simulink model "L0401"  (Simulink 9.1)
settings: Solver=ode5  StartTime=0.0  StopTime=100  FixedStep=0.001  RelTol=1e-3
values from neighbouring files (symbols this model uses):
  c = input('Damping parameter c= ')    [vehicle.m]
  hole_depth = 0.15    [vehicle.m]
  k = input('Spring stiffness k= ')    [vehicle.m]
  m = 1000    [vehicle.m]
  t1 = hole_start/v    (= 22.5)    [vehicle.m]
  t2 = (hole_start + hole_width)/v    (= 22.55)    [vehicle.m]
settings Model: Creator=Asus  LastModifiedBy=Asus
settings DataIOCC: SaveFormat=Dataset
settings OptimizationCC: LifeSpan=auto
settings DebuggingCC: UnderspecifiedInitializationDetection=Simplified  MergeDetectMultiDrivingBlocksExec=error  SFUnexpectedBacktrackingDiag=error  SFNoUnconditionalDefaultTransitionDiag=error  SFExecutionAtInitializationDiag=warning
settings HardwareCC: ProdBitPerPointer=64  ProdBitPerSizeT=64  ProdBitPerPtrDiffT=64  ProdLargestAtomicFloat=Float  ProdIntDivRoundTo=Zero  ProdEndianess=LittleEndian  ProdWordSize=64  ProdHWDeviceType=Intel->x86-64 (Windows64)
settings ModelReferenceCC: PropagateSignalLabelsOutOfModel=on
settings CodeAppCC: StateflowObjectComments=off
settings GRTTargetCC: TargetLangStandard=C99 (ISO)  CombineOutputUpdateFcns=on  GRTInterface=off
settings ConfigComp: CovMetricSettings=dwe  CovHtmlReporting=off  CovSaveCumulativeToWorkspaceVar=off  CovSaveSingleToWorkspaceVar=off  CovExternalEMLEnable=on

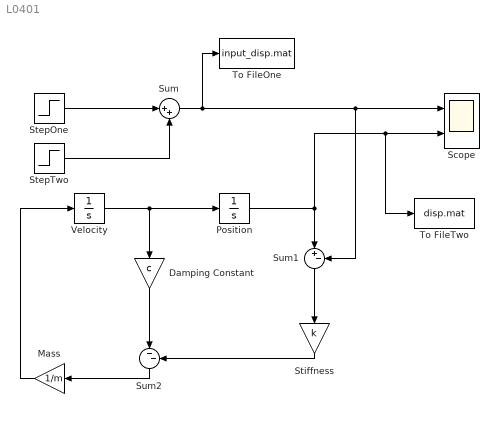
== system L0401 ==
  Damping Constant : Gain  Gain=c
  Mass : Gain  Gain=1/m
  Position : Integrator
  Scope : Scope  NumInputPorts=2
  StepOne : Step  Time=t1  After=-hole_depth  SampleTime=0.001
  StepTwo : Step  Time=t2  After=hole_depth  SampleTime=0.001
  Stiffness : Gain  Gain=k
  Sum : Sum  Inputs=|++
  Sum1 : Sum  Inputs=|+-
  Sum2 : Sum  Inputs=|--
  To FileOne : ToFile  Filename=input_disp.mat  MatrixName=input_disp  SaveFormat=Timeseries
  To FileTwo : ToFile  Filename=disp.mat  MatrixName=disp  SaveFormat=Timeseries
  Velocity : Integrator
  wires:
  StepTwo/1 -> Sum/2
  StepOne/1 -> Sum/1
  Velocity/1 -> Damping Constant/1, Position/1
  Sum/1 -> To FileOne/1, Sum1/2, Scope/1
  Position/1 -> Scope/2, To FileTwo/1, Sum1/1
  Sum1/1 -> Stiffness/1
  Stiffness/1 -> Sum2/2
  Damping Constant/1 -> Sum2/1
  Sum2/1 -> Mass/1
  Mass/1 -> Velocity/1
